simulink model "Manipulator_PDControl_InteractionControlHybrImpControl_for"  (R2020b)
settings: Solver=FixedStepAuto  StartTime=0.0  StopTime=t_final  FixedStep=dt  RelTol=1e-3
values from neighbouring files (symbols this model uses):
  dq_0 = 0.1 *[ 0  -1  0]    [Initialization.m]
  dt = 1.00e-03    (= 0.001)    [Initialization.m]
  ikInitGuessSim = ikInitGuess    [generateTrajectory.m]
  q_0 = [0;-0.9;2.7]    [Initialization.m]
  waypointAccels = zeros(size(waypointVels))    [generateTrajectory.m]
  waypoints = initPosition +              [0 0 0 ; 0 -a -a ; 0 0 -2*a; 0 a -a ; 0 0 0]'    [generateTrajectory.m]
  waypointVels = 0.1 *[ 0  -1  0 ... (first row only)    [generateTrajectory.m]
libraries: simulink x4, robotcorelib x2, robotmaniplib x1
settings Model: Creator=m2aali  LastModifiedBy=Kons
settings DataIOCC: LoggingToFile=on

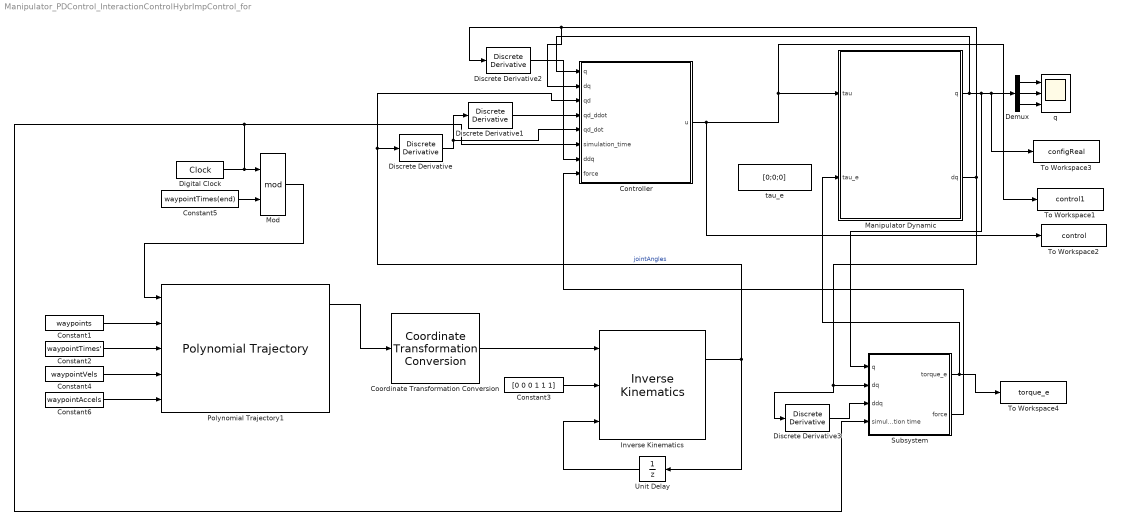
== system Manipulator_PDControl_InteractionControlHybrImpControl_for ==
  Constant1 : Constant  Value=waypoints  VectorParams1D=off  SampleTime=-1
  Constant2 : Constant  Value=waypointTimes'  VectorParams1D=off  SampleTime=-1
  Constant3 : Constant  Value=[0 0 0 1 1 1]  VectorParams1D=off
  Constant4 : Constant  Value=waypointVels  VectorParams1D=off  SampleTime=-1
  Constant5 : Constant  Value=waypointTimes(end)
  Constant6 : Constant  Value=waypointAccels  VectorParams1D=off  SampleTime=-1
  Controller : Subsystem
  Coordinate Transformation Conversion : robotcorelib/Coordinate Transformation Conversion  InputRepresentation=Translation Vector  InputEulerSequence=ZYX  ShowTrVecInputPort=on  OutputRepresentation=Homogeneous Transformation  OutputEulerSequence=ZYX  ShowTrVecOutputPort=on  SimulateUsing=Code generation
      settings: SourceProductBaseCode=NV,RO,RR,UV
  Demux : Demux  Outputs=3
  Digital Clock : DigitalClock  SampleTime=dt
  Discrete Derivative : simulink/Discrete/Discrete Derivative  gainval=1.0  ICPrevScaledInput=[-0.000001274337461;-0.900000000000479;2.699999999999876]*1000  OutMin=[]  OutMax=[]  OutDataType=fixdt(1, 16)  OutScaling=2^-10  DoSatur=off
  Discrete Derivative1 : simulink/Discrete/Discrete Derivative  gainval=1.0  ICPrevScaledInput="[ 0 ; 0;  0]"  OutMin=[]  OutMax=[]  OutDataType=fixdt(1, 16)  OutScaling=2^-10  DoSatur=off
  Discrete Derivative2 : simulink/Discrete/Discrete Derivative  gainval=1.0  ICPrevScaledInput="[ 0 ; 0;  0]"  OutMin=[]  OutMax=[]  OutDataType=fixdt(1, 16)  OutScaling=2^-10  DoSatur=off
  Discrete Derivative3 : simulink/Discrete/Discrete Derivative  gainval=1.0  ICPrevScaledInput="[ 0 ; 0;  0]"  OutMin=[]  OutMax=[]  OutDataType=fixdt(1, 16)  OutScaling=2^-10  DoSatur=off
  Inverse Kinematics : robotmaniplib/Inverse Kinematics  RigidBodyTree=robot  EndEffector=Link_EE  ShowInfo=on  SolverName=BFGS Gradient Projection  EnforceJointLimits=on  MaxIterations=1500  MaxTime=10  GradientTolerance=1e-7  SolutionTolerance=1e-6  StepTolerance=1e-14  ErrorChangeTolerance=1e-12  UseErrorDamping=on  DampingBias=0.0025  SimulateUsing=Code generation
  Manipulator Dynamic : Subsystem
  Mod : Math  Operator=mod  SignedPower=on  SaturateOnIntegerOverflow=on
  Polynomial Trajectory1 : robotcorelib/Polynomial Trajectory  WaypointSource=External  Waypoints=[ 0, 2, 1, 5, 0; -1, 3, 1, 4, 4 ]  TimePoints=[ 0, 1, 2, 3, 4 ]  TimeInterval=[ 1, 4 ]  Method=Quintic Polynomial  ParameterSource=External  VelocityBoundaryCondition=zeros( 2, 5 )  AccelerationBoundaryCondition=zeros( 2, 5 )  SimulateUsing=Code generation
  Subsystem : Subsystem
  To Workspace1 : ToWorkspace  VariableName=control1  SaveFormat=Timeseries  SampleTime=-1
  To Workspace2 : ToWorkspace  VariableName=control  SaveFormat=Timeseries  SampleTime=-1
  To Workspace3 : ToWorkspace  VariableName=configReal  SaveFormat=Timeseries  SampleTime=-1
  To Workspace4 : ToWorkspace  VariableName=torque_e  SaveFormat=Timeseries  SampleTime=-1
  Unit Delay : UnitDelay  InitialCondition=ikInitGuessSim  SampleTime=-1  HasFrameUpgradeWarning=on
  q : Scope  NumInputPorts=3
  tau_e : Constant  Value=[0;0;0]
  wires:
  Manipulator Dynamic/2(dq) -> Discrete Derivative3/1, Subsystem/2(dq), Discrete Derivative2/1, Controller/2(dq)
  Controller/1(u) -> To Workspace2/1, To Workspace1/1, Manipulator Dynamic/1(tau)
  Demux/1 -> q/1
  Demux/2 -> q/2
  Demux/3 -> q/3
  Digital Clock/1 -> Controller/6(simulation_time), Subsystem/4(simulation time), Mod/1
  Mod/1 -> Polynomial Trajectory1/1
  Constant5/1 -> Mod/2
  Polynomial Trajectory1/1 -> Coordinate Transformation Conversion/1
  Inverse Kinematics/1 -> Unit Delay/1, Controller/3(qd), Discrete Derivative/1  "jointAngles"
  Unit Delay/1 -> Inverse Kinematics/3
  Constant3/1 -> Inverse Kinematics/2
  Coordinate Transformation Conversion/1 -> Inverse Kinematics/1
  Discrete Derivative1/1 -> Controller/4(qd_ddot)
  Discrete Derivative/1 -> Discrete Derivative1/1, Controller/5(qd_dot)
  Constant1/1 -> Polynomial Trajectory1/2
  Constant2/1 -> Polynomial Trajectory1/3
  Constant4/1 -> Polynomial Trajectory1/4
  Constant6/1 -> Polynomial Trajectory1/5
  Manipulator Dynamic/1(q) -> Subsystem/1(q), To Workspace3/1, Demux/1, Controller/1(q)
  Discrete Derivative2/1 -> Controller/7(ddq)
  Discrete Derivative3/1 -> Subsystem/3(ddq)
  Subsystem/1(torque_e) -> Manipulator Dynamic/2(tau_e), To Workspace4/1
  Subsystem/2(force) -> Controller/8(force)

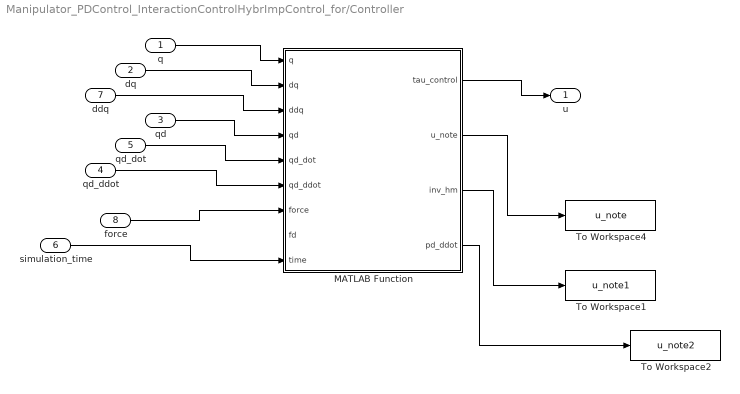
== system Manipulator_PDControl_InteractionControlHybrImpControl_for/Controller ==
  q : Inport
  dq : Inport  Port=2
  qd : Inport  Port=3
  qd_ddot : Inport  Port=4
  qd_dot : Inport  Port=5
  simulation_time : Inport  Port=6
  ddq : Inport  Port=7
  force : Inport  Port=8
  MATLAB Function : MATLAB Function  TreatAsAtomicUnit=on
  To Workspace1 : ToWorkspace  VariableName=u_note1  SaveFormat=Timeseries  SampleTime=-1
  To Workspace2 : ToWorkspace  VariableName=u_note2  SaveFormat=Timeseries  SampleTime=-1
  To Workspace4 : ToWorkspace  VariableName=u_note  SaveFormat=Timeseries  SampleTime=-1
  u : Outport
  wires:
  dq/1 -> MATLAB Function/2(dq)
  MATLAB Function/1(tau_control) -> u/1
  qd/1 -> MATLAB Function/4(qd)
  q/1 -> MATLAB Function/1(q)
  qd_ddot/1 -> MATLAB Function/6(qd_ddot)
  qd_dot/1 -> MATLAB Function/5(qd_dot)
  simulation_time/1 -> MATLAB Function/9(time)
  ddq/1 -> MATLAB Function/3(ddq)
  force/1 -> MATLAB Function/7(force)
  MATLAB Function/2(u_note) -> To Workspace4/1
  MATLAB Function/3(inv_hm) -> To Workspace1/1
  MATLAB Function/4(pd_ddot) -> To Workspace2/1

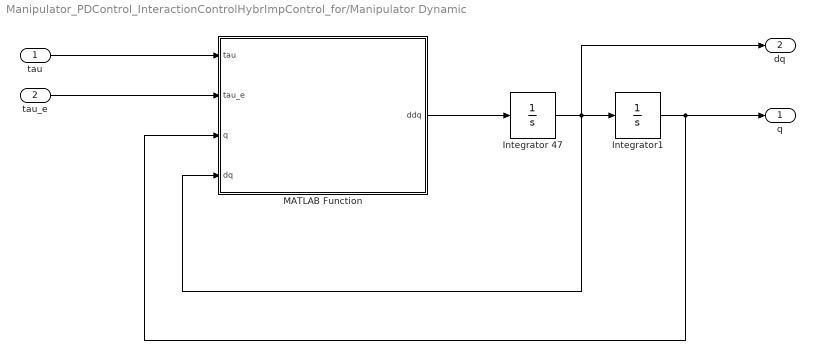
== system Manipulator_PDControl_InteractionControlHybrImpControl_for/Manipulator Dynamic ==
  tau : Inport
  tau_e : Inport  Port=2
  Integrator 47 : Integrator  InitialCondition=dq_0
  Integrator1 : Integrator  InitialCondition=q_0
  MATLAB Function : MATLAB Function  TreatAsAtomicUnit=on
  q : Outport
  dq : Outport  Port=2
  wires:
  MATLAB Function/1(ddq) -> Integrator 47/1
  tau/1 -> MATLAB Function/1(tau)
  tau_e/1 -> MATLAB Function/2(tau_e)
  Integrator1/1 -> q/1, MATLAB Function/3(q)
  Integrator 47/1 -> dq/1, MATLAB Function/4(dq), Integrator1/1

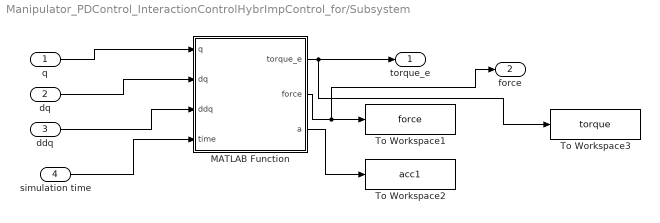
== system Manipulator_PDControl_InteractionControlHybrImpControl_for/Subsystem ==
  q : Inport
  dq : Inport  Port=2
  ddq : Inport  Port=3
  simulation time : Inport  Port=4
  MATLAB Function : MATLAB Function  TreatAsAtomicUnit=on
  To Workspace1 : ToWorkspace  VariableName=force  SaveFormat=Timeseries  SampleTime=-1
  To Workspace2 : ToWorkspace  VariableName=acc1  SaveFormat=Timeseries  SampleTime=-1
  To Workspace3 : ToWorkspace  VariableName=torque  SaveFormat=Timeseries  SampleTime=-1
  torque_e : Outport
  force : Outport  Port=2
  wires:
  q/1 -> MATLAB Function/1(q)
  dq/1 -> MATLAB Function/2(dq)
  ddq/1 -> MATLAB Function/3(ddq)
  MATLAB Function/1(torque_e) -> To Workspace3/1, torque_e/1
  MATLAB Function/3(a) -> To Workspace2/1
  MATLAB Function/2(force) -> force/1, To Workspace1/1
  simulation time/1 -> MATLAB Function/4(time)

== matlab function Manipulator_PDControl_InteractionControlHybrImpControl_for/Controller/MATLAB Function ==
  data: q input; dq input; ddq input; tau_control output; qd input; qd_dot input; qd_ddot input; force input; fd input; time input; u_note output; inv_hm output; pd_ddot output
function [tau_control, u_note,inv_hm,pd_ddot]  = fcn(q, dq, ddq, qd, qd_dot, qd_ddot,force,fd,...
                                                                  time)
% reset first qd_ddot
if (time < 0.003)
    qd_ddot = [0;0;0];
    qd_dot = [0;0;0];
    ddq = [0;0;0];
end


%% Joint Space variables

q1 = q(1);
q2 = q(2);
q3 = q(3);

dq1 = dq(1);
dq2 = dq(2);
dq3 = dq(3);

%% general physical parameters

l1 = 0.6731;
l2 = 0.432;
l3 = 0.434;
lc2 = 0.216;
lc3 = 0.164;
m2 = 15.46;
m3 = 9.55;
J = 0.302;

%% Inertia Matrix Parameters

J1 = m3 * lc3^2;
J12 = (m2 * lc2^2) + (m3 * l2^2);
J13 = l2 * lc3 * m3;


h11 = J + J1 * (sin(q2 + q3))^2 + J12 * (cos(q2))^2 + 2 * J13 * cos(q2) * sin(q2+q3);
h22 = J1 + J12 + 2 * J13 * sin(q3);
h23 = J1 + J13 * sin(q3);
h32 = h23;
h33 = J1;

H = [h11, 0 ,0 ;
    0 , h22, h23;
    0 , h32, h33];

%% Coriolis Matrix Parameters

c12_1 = J1 * sin(2 * (q1 + q2)) - J12 * sin(2 * q2) + 2 * J13 * cos(2 * q2 +q3);
c13_1 = J1 * sin(2 * (q2 + q3)) + 2 * J13 * cos(q2) * cos(q2 + q3);
c11_2 = (1/2) * (-J1 * sin(2 * (q2 + q3)) + J12 * sin(2 * q2) - 2 * J13 * cos(2 * q2 + q3));
c22_2 = 2 * J13 * cos(q3);
c23_2 = J13 * cos(q3);
c22_3 = -J13 * cos(q3) * dq2;
c11_3 = (-1/2) * (J1 * sin(2 * (q2 + q3)) + J13 * cos(q2) * cos(q2 + q3));

C = [0, c12_1 * dq1, c13_1 * dq3;
    c11_2 * dq1, 0 , c22_2 * dq2 + c23_2 * dq3;
    c11_3 * dq1, c22_3 * dq2, 0];

%% Vector of Potential Forces Parameters

g = 9.81;

g21 = -g * (lc3 * m3 * sin(q2 + q3) + lc2 * m2 * cos(q2) + l2 * m3 * cos(q2));
g31 = -g * (lc3 * m3 * sin(q2 + q3));

G = [0;
    g21;
    g31];


%% get Jacobians
J = jacobian(q);
dJ = dJacobian(q,dq);

%% convert to task space
Hp = inv(J') * H * inv(J);
Cp = inv(J') * C * inv(J) - Hp * dJ * inv(J);
Gp = inv(J') * G;

%% desired behaviour 
Hm = [1 0 0; 0 1 0; 0 0 1];
Dm = [20 0 0; 0 20 0; 0 0 20];
Km = [0 0 0; 0 0  0; 0 0 0];

%% get postion and its derivs
p = fwdKin(q);
dp = J * dq;
ddp = dJ * dq + J * ddq;

%% get desired postion and its derivs
pd = fwdKin(qd);
pd_dot = jacobian(qd) * qd_dot;
pd_ddot = dJacobian(qd,qd_dot) * qd_dot + jacobian(qd) * qd_ddot;

%% define des force
total_time = 10;
f_magn = 3.15;
alpha = 0 + (2*pi / total_time) * time;
fy = f_magn * cos(alpha);
fz = f_magn * sin(alpha);
fd = [0;fy;fz];
%% define u note, velocity control mode

u_note = inv(Hm) * (-Dm * (dp) - Km*(p) + force - fd);
inv_hm = inv(Hm);
%% define tau_control

tau_control = J' * (Hp * u_note + Cp * dp + Gp - force);


function [X] = fwdKin(Q)
    s1 = sin(Q(1, :));
    c1 = cos(Q(1, :));
    s2 = sin(Q(2, :));
    c2 = cos(Q(2, :));
    s23 = sin(Q(2, :) + Q(3, :));
    c23 = cos(Q(2, :) + Q(3, :));
    l = [0.6731; 0.432; 0.434];
    
    X = zeros(3,1)
    X(1, :) = c1.*(l(2)*c2 + l(3)*s23);
    X(2, :) = s1.*(l(2)*c2 + l(3)*s23);
    X(3, :) = l(1) - l(2)*s2 + l(3)*c23;

function dJ = dJacobian(Q, dQ)
    l = [0.6731; 0.432; 0.434];
    s1 = sin(Q(1));
    c1 = cos(Q(1));
    s2 = sin(Q(2));
    c2 = cos(Q(2));
    s23 = sin(Q(2) + Q(3));
    c23 = cos(Q(2) + Q(3));

    % dJi derivative of each element of Jacobian wrt i-th variable            
    %--- 1 ---
    dJ1 = [-c1*(l(2)*c2 + l(3)*s23), -s1*(-l(2)*s2 + l(3)*c23), -l(3)*s1*c23;...
           -s1*(l(2)*c2 + l(3)*s23),  c1*(-l(2)*s2 + l(3)*c23),  l(3)*c1*c23;...
           0, 0, 0];
    %--- 2 ---   
    dJ2 = [-s1*(-l(2)*s2 + l(3)*c23), -c1*(l(2)*c2 + l(3)*s23), -l(3)*c1*s23;...
            c1*(-l(2)*s2 + l(3)*c23), -s1*(l(2)*c2 + l(3)*s23), -l(3)*s1*s23;...
            0, l(2)*s2 - l(3)*c23, -l(3)*c23];

    %--- 3 ---
    dJ3 = -l(3)*[ s1*c23, c1*s23, c1*s23;...
                 -c1*c23, s1*s23, s1*s23;...
                 0, c23, c23];
    %--- dJ ---
    dJ = dJ1*dQ(1) + dJ2*dQ(2) + dJ3*dQ(3);

function [J] = jacobian(q)

l = [0.6731; 0.432; 0.434];
s1 = sin(q(1));
c1 = cos(q(1));
s2 = sin(q(2));
c2 = cos(q(2));
s23 = sin(q(2) + q(3));
c23 = cos(q(2) + q(3));

J = zeros(3,3);

J(1, 1) = -s1*( l(2)*c2 + l(3)*s23);
J(1, 2) =  c1*(-l(2)*s2 + l(3)*c23);
J(1, 3) = l(3)*c1*c23;

J(2, 1) = c1*( l(2)*c2 + l(3)*s23);
J(2, 2) = s1*(-l(2)*s2 + l(3)*c23);
J(2, 3) = l(3)*s1*c23;

J(3, 2) = -l(2)*c2 - l(3)*s23;
J(3, 3) = -l(3)*s23;

== matlab function Manipulator_PDControl_InteractionControlHybrImpControl_for/Manipulator Dynamic/MATLAB Function ==
  data: tau input; tau_e input; q input; ddq output; dq input
function ddq = DynamicModel( tau, tau_e, q, dq)
%%%%%
% 3-DOF Puma-560 Dynamic Model Function
% H(q)* ddq + C(q) * dq + G = tau + tau_e
% q is 3*1 vector of joint variables (radian)
% H(q) is the inertia matrix
% C(q) is the matrix of Coriolis and centrifugal forces
% G(q) is  the vector of potential forces Parameters
% tau is control torque 
% tau_e is the external torque due to the interaction with the environment
%%%%%

%% Joint Space variables

q1 = q(1);
q2 = q(2);
q3 = q(3);

dq1 = dq(1);
dq2 = dq(2);
dq3 = dq(3);

%% general physical parameters

l1 = 0.6731;
l2 = 0.432;
l3 = 0.434;
lc2 = 0.216;
lc3 = 0.164;
m2 = 15.46;
m3 = 9.55;
J = 0.302;

%% Inertia Matrix Parameters

J1 = m3 * lc3^2;
J12 = (m2 * lc2^2) + (m3 * l2^2);
J13 = l2 * lc3 * m3;


h11 = J + J1 * (sin(q2 + q3))^2 + J12 * (cos(q2))^2 + 2 * J13 * cos(q2) * sin(q2+q3);
h22 = J1 + J12 + 2 * J13 * sin(q3);
h23 = J1 + J13 * sin(q3);
h32 = h23;
h33 = J1;

H = [h11, 0 ,0 ;
    0 , h22, h23;
    0 , h32, h33];

%% Coriolis Matrix Parameters

c12_1 = J1 * sin(2 * (q1 + q2)) - J12 * sin(2 * q2) + 2 * J13 * cos(2 * q2 +q3);
c13_1 = J1 * sin(2 * (q2 + q3)) + 2 * J13 * cos(q2) * cos(q2 + q3);
c11_2 = (1/2) * (-J1 * sin(2 * (q2 + q3)) + J12 * sin(2 * q2) - 2 * J13 * cos(2 * q2 + q3));
c22_2 = 2 * J13 * cos(q3);
c23_2 = J13 * cos(q3);
c22_3 = -J13 * cos(q3) * dq2;
c11_3 = (-1/2) * (J1 * sin(2 * (q2 + q3)) + J13 * cos(q2) * cos(q2 + q3));

C = [0, c12_1 * dq1, c13_1 * dq3;
    c11_2 * dq1, 0 , c22_2 * dq2 + c23_2 * dq3;
    c11_3 * dq1, c22_3 * dq2, 0];

%% Vector of Potential Forces Parameters

g = 9.81;

g21 = -g * (lc3 * m3 * sin(q2 + q3) + lc2 * m2 * cos(q2) + l2 * m3 * cos(q2));
g31 = -g * (lc3 * m3 * sin(q2 + q3));

G = [0;
    g21;
    g31];

%% Function output

ddq = inv(H)*(tau + tau_e - C * dq - G);

== matlab function Manipulator_PDControl_InteractionControlHybrImpControl_for/Subsystem/MATLAB Function ==
  data: q input; torque_e output; force output; dq input; ddq input; a output; time input
function [torque_e,force,a]  = fcn(q,dq, ddq, time)

if (time < 0.003)
    ddq = [0;0;0];
end

J = jacobian(q);
dJ = dJacobian(q, dq);

pos = fwdKin(q);
v = J * dq;
a = dJ * dq + J * ddq;

M = [0 0 0; 0 0 0 ; 0 0 0];
D = [100 0 0; 0 0 0 ; 0 0 0];
K = [0 0 0; 0 0 0 ; 0 0 0];

env_nom = [0.691185378094064;0;0.912891515862273];
env_nom = env_nom - [0.05;0;0];
%% calculate force
force = -(M*a + D*v + K*(pos - env_nom));

torque_e = J' * force;

% if (pos(1) < env_nom(1))
%     torque_e = [0;0;0];
%     force = [0;0;0];
% end


function [X] = fwdKin(Q)
    s1 = sin(Q(1, :));
    c1 = cos(Q(1, :));
    s2 = sin(Q(2, :));
    c2 = cos(Q(2, :));
    s23 = sin(Q(2, :) + Q(3, :));
    c23 = cos(Q(2, :) + Q(3, :));
    l = [0.6731; 0.432; 0.434];
    
    X = zeros(3,1)
    X(1, :) = c1.*(l(2)*c2 + l(3)*s23);
    X(2, :) = s1.*(l(2)*c2 + l(3)*s23);
    X(3, :) = l(1) - l(2)*s2 + l(3)*c23;

function dJ = dJacobian(Q, dQ)
    l = [0.6731; 0.432; 0.434];
    s1 = sin(Q(1));
    c1 = cos(Q(1));
    s2 = sin(Q(2));
    c2 = cos(Q(2));
    s23 = sin(Q(2) + Q(3));
    c23 = cos(Q(2) + Q(3));

    % dJi derivative of each element of Jacobian wrt i-th variable            
    %--- 1 ---
    dJ1 = [-c1*(l(2)*c2 + l(3)*s23), -s1*(-l(2)*s2 + l(3)*c23), -l(3)*s1*c23;...
           -s1*(l(2)*c2 + l(3)*s23),  c1*(-l(2)*s2 + l(3)*c23),  l(3)*c1*c23;...
           0, 0, 0];
    %--- 2 ---   
    dJ2 = [-s1*(-l(2)*s2 + l(3)*c23), -c1*(l(2)*c2 + l(3)*s23), -l(3)*c1*s23;...
            c1*(-l(2)*s2 + l(3)*c23), -s1*(l(2)*c2 + l(3)*s23), -l(3)*s1*s23;...
            0, l(2)*s2 - l(3)*c23, -l(3)*c23];

    %--- 3 ---
    dJ3 = -l(3)*[ s1*c23, c1*s23, c1*s23;...
                 -c1*c23, s1*s23, s1*s23;...
                 0, c23, c23];
    %--- dJ ---
    dJ = dJ1*dQ(1) + dJ2*dQ(2) + dJ3*dQ(3);

function [J] = jacobian(q)

l = [0.6731; 0.432; 0.434];
s1 = sin(q(1));
c1 = cos(q(1));
s2 = sin(q(2));
c2 = cos(q(2));
s23 = sin(q(2) + q(3));
c23 = cos(q(2) + q(3));

J = zeros(3,3);

J(1, 1) = -s1*( l(2)*c2 + l(3)*s23);
J(1, 2) =  c1*(-l(2)*s2 + l(3)*c23);
J(1, 3) = l(3)*c1*c23;

J(2, 1) = c1*( l(2)*c2 + l(3)*s23);
J(2, 2) = s1*(-l(2)*s2 + l(3)*c23);
J(2, 3) = l(3)*s1*c23;

J(3, 2) = -l(2)*c2 - l(3)*s23;
J(3, 3) = -l(3)*s23;
